simulink model "ControlSystem"  (R2020a)
settings: Solver=ode45  StartTime=0  StopTime=50  RelTol=1e-3  EnableMultiTasking=on
libraries: Solver_SF x2, simulink_extras x2, mpcadaslib x1, simulink x1
settings Model: ExtModeTrigMode=oneshot  ExtModeArmWhenConnect=off  Creator=dhall  LastModifiedBy=Zeng baiming
settings DataIOCC: SaveFormat=Array  SignalLoggingSaveFormat=ModelDataLogs  ReturnWorkspaceOutputs=off  SignalLoggingName=sigsOut
settings OptimizationCC: BooleanDataType=off  LocalBlockOutputs=off  InitFltsAndDblsToZero=on  LifeSpan=inf
settings DebuggingCC: SaveWithParameterizedLinksMsg=none  UnderspecifiedInitializationDetection=Classic  MergeDetectMultiDrivingBlocksExec=none  SignalResolutionControl=TryResolveAllWithWarning  MultiTaskDSMMsg=warning  MultiTaskCondExecSysMsg=none  FcnCallInpInsideContextMsg=warning  StateNameClashWarn=warning  SFUnexpectedBacktrackingDiag=warning  SFNoUnconditionalDefaultTransitionDiag=warning  SFExecutionAtInitializationDiag=none  ArithmeticOperatorsInVariantConditions=warning
settings HardwareCC: ProdBitPerPointer=32  ProdBitPerSizeT=32  ProdBitPerPtrDiffT=32  ProdLargestAtomicFloat=None  ProdIntDivRoundTo=Undefined  ProdEndianess=Unspecified  ProdWordSize=32  ProdHWDeviceType=32-bit Generic  TargetUnknown=on
settings ModelReferenceCC: PropagateSignalLabelsOutOfModel=off
settings SFSimCC: SimUseLocalCustomCode=off  CustomCodeUndefinedFunction=UseInterfaceOnly
settings RTWCC: RTWUseLocalCustomCode=off
settings CodeAppCC: StateflowObjectComments=on
settings GRTTargetCC: TargetFcnLib=ansi_tfl_tmw.mat  TargetLangStandard=C89/C90 (ANSI)  CompOptLevelCompliant=off  CombineOutputUpdateFcns=off  GRTInterface=on
settings ConfigComp: CovMetricSettings=dw  CovHtmlReporting=on  CovSaveCumulativeToWorkspaceVar=on  CovSaveSingleToWorkspaceVar=on  CovExternalEMLEnable=off

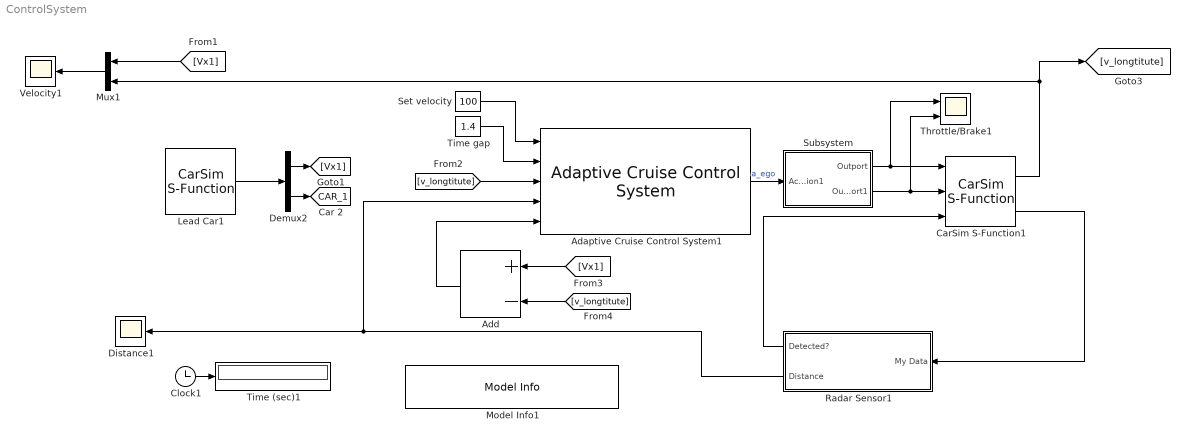
== system ControlSystem ==
  Adaptive Cruise Control System1 : mpcadaslib/Adaptive Cruise Control System  EgoModel=tf(1,[0.5,1,0])  InitialEgoVelocity=20  DefaultSpacing=10  MaxVelocity=50  MinAcceleration=-3  amin_ext=off  MaxAcceleration=2  amax_ext=off  Ts=0.1  PredictionHorizon=30  ControllerBehavior=0.5  suboptimal=off  maxiter=10  datatypeopt=double  optmode=off  trackmode=off
  Add : Sum  Inputs=+-
  CarSim S-Function1 : Solver_SF/CarSim S-Function  Priority=1  SIMFILE=Radar_Acc_ExtSen_Car_2.sim
  Clock1 : Clock
  Demux2 : Demux  Outputs=[1 3]
      settings: DisplayOption=none
  Distance1 : Scope
  Lead Car1 : Solver_SF/CarSim S-Function  Priority=1  SIMFILE=Radar_Acc_ExtSen_Car_1.sim
  Model Info1 : simulink/Model-Wide Utilities/Model Info  Frame=on  DisplayStringWithTags=Multi Vehicle Run Adaptive Cruise Control Model  HorizontalTextAlignment=Center  LeftAlignmentValue=0.5
  Mux1 : Mux  Inputs=2
  Radar Sensor1 : Subsystem  mask{S_ANGLE=10, S_DISTANCE=70}
      mask prompts: S_ANGLE "View Angle (deg)"; S_DISTANCE "Distance Range (m)"
      mask help:
      | An example of a radar sensor. It can detect the distance between the sensor and another object according its position (Xo, Yo).
      |
      | Input parameters are View Angle(deg) and radar detectable distance(m).
      mask init:
      | d_ang= str2double(S_ANGLE)/2;
      | set_param([gcb '/View Angle'], 'Threshold', sprintf('%0.2f', d_ang));
      | set_param([gcb '/L-Radar'], 'Value', S_DISTANCE);
  Set velocity : Constant  Value=100  SampleTime=0.1
  Subsystem : Subsystem
  Throttle/Brake1 : Scope  NumInputPorts=2
  Time (sec)1 : Display
      settings: Format=bank  Decimation=100
  Time gap : Constant  Value=1.4  SampleTime=0.1
  Velocity1 : Scope
  tag scope: CAR_1=global
  wires:
  Lead Car1/1 -> Demux2/1
  [Vx1] -> Mux1/1
  CarSim S-Function1/1 -> [v_longtitute], Mux1/2
  Radar Sensor1/2(Distance) -> Distance1/1, Adaptive Cruise Control System1/4
  Demux2/1 -> [Vx1]
  Demux2/2 -> [CAR_1]
  Mux1/1 -> Velocity1/1
  CarSim S-Function1/2 -> Radar Sensor1/1(My Data)
  Subsystem/1(Outport) -> Throttle/Brake1/1, CarSim S-Function1/1
  Clock1/1 -> Time (sec)1/1
  Subsystem/2(Outport1) -> Throttle/Brake1/2, CarSim S-Function1/2
  Radar Sensor1/1(Detected?) -> CarSim S-Function1/3
  Set velocity/1 -> Adaptive Cruise Control System1/1
  Time gap/1 -> Adaptive Cruise Control System1/2
  Adaptive Cruise Control System1/1 -> Subsystem/1(Acceleration1)  "a_ego"
  [v_longtitute] -> Adaptive Cruise Control System1/3
  [Vx1] -> Add/1
  [v_longtitute] -> Add/2
  Add/1 -> Adaptive Cruise Control System1/5

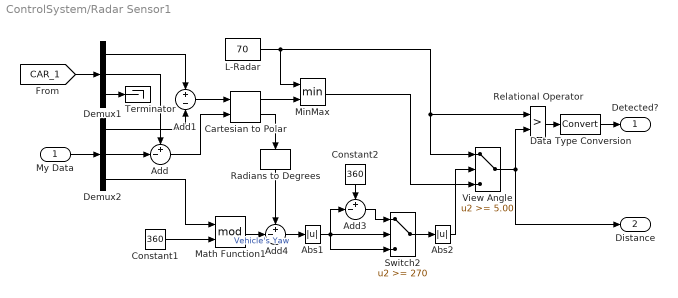
== system ControlSystem/Radar Sensor1 ==
  My Data : Inport
  Abs1 : Abs
  Abs2 : Abs
  Add : Sum  Inputs=+-|
  Add1 : Sum  Inputs=+-
  Add3 : Sum  Inputs=+-|
  Add4 : Sum  Inputs=+-|
  Cartesian to Polar : simulink_extras/Transformations/Cartesian to Polar
  Constant1 : Constant  Value=360
  Constant2 : Constant  Value=360
  Data Type Conversion : DataTypeConversion  RndMeth=Zero
  Demux1 : Demux  Outputs=3
      settings: DisplayOption=none
  Demux2 : Demux  Outputs=3
      settings: DisplayOption=none
  L-Radar : Constant  Value=70
  Math Function1 : Math  Operator=mod  SignedPower=on  SaturateOnIntegerOverflow=on
  MinMax : MinMax  Inputs=2  InputSameDT=on  SaturateOnIntegerOverflow=on
  Radians to Degrees : simulink_extras/Transformations/Radians to Degrees
  Relational Operator : RelationalOperator  Operator=>  OutDataTypeStr=boolean  RndMeth=Nearest
  Switch2 : Switch  Threshold=270
  Terminator : Terminator
  View Angle : Switch  Threshold=5.00
  Detected? : Outport
  Distance : Outport  Port=2
  wires:
  Cartesian to Polar/2 -> Radians to Degrees/1
  Cartesian to Polar/1 -> MinMax/2
  Radians to Degrees/1 -> Add4/1
  Data Type Conversion/1 -> Detected?/1
  Relational Operator/1 -> Data Type Conversion/1
  View Angle/1 -> Relational Operator/2, Distance/1
  Abs2/1 -> View Angle/2
  Switch2/1 -> Abs2/1
  MinMax/1 -> View Angle/3
  L-Radar/1 -> Relational Operator/1, View Angle/1, MinMax/1
  Constant2/1 -> Add3/1
  Add3/1 -> Switch2/1
  Abs1/1 -> Switch2/3, Add3/2, Switch2/2
  Add4/1 -> Abs1/1
  Math Function1/1 -> Add4/2  "Vehicle's Yaw"
  [CAR_1] -> Demux1/1
  My Data/1 -> Demux2/1
  Demux1/3 -> Terminator/1
  Demux1/2 -> Add/1
  Demux2/2 -> Add/2
  Demux1/1 -> Add1/1
  Demux2/1 -> Add1/2
  Add1/1 -> Cartesian to Polar/1
  Add/1 -> Cartesian to Polar/2
  Constant1/1 -> Math Function1/2
  Demux2/3 -> Math Function1/1

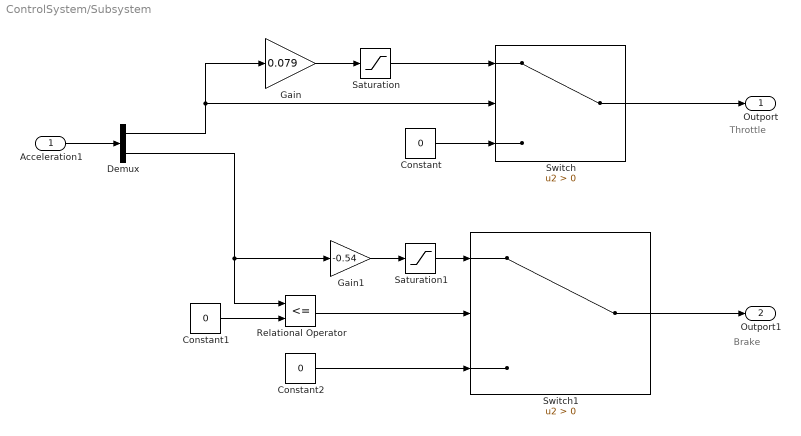
== system ControlSystem/Subsystem ==
  note: Brake
  note: Throttle
  Acceleration1 : Inport
  Constant : Constant  Value=0
  Constant1 : Constant  Value=0
  Constant2 : Constant  Value=0
  Demux : Demux  Outputs=2
  Gain : Gain  Gain=0.079
  Gain1 : Gain  Gain=-0.54
  Relational Operator : RelationalOperator  Operator=<=  OutDataTypeStr=boolean  RndMeth=Simplest
  Saturation : Saturate
  Saturation1 : Saturate  UpperLimit=3
  Switch : Switch  Criteria=u2 > Threshold
  Switch1 : Switch  Criteria=u2 > Threshold
  Outport : Outport
  Outport1 : Outport  Port=2
  wires:
  Switch1/1 -> Outport1/1
  Saturation1/1 -> Switch1/1
  Saturation/1 -> Switch/1
  Acceleration1/1 -> Demux/1
  Constant1/1 -> Relational Operator/2
  Switch/1 -> Outport/1
  Gain/1 -> Saturation/1
  Gain1/1 -> Saturation1/1
  Relational Operator/1 -> Switch1/2
  Constant2/1 -> Switch1/3
  Demux/2 -> Gain1/1, Relational Operator/1
  Constant/1 -> Switch/3
  Demux/1 -> Switch/2, Gain/1
